simulink model "UDE_quadrotor"  (R2017b)
settings: Solver=ode4  StartTime=0.0  StopTime=40  FixedStep=0.001  RelTol=1e-3
InitFcn:
  | initial_conditions_and_parameters;
values from neighbouring files (symbols this model uses):
  psi_initial = 0.0    (= 0)    [Parameters_and_initial_conditions.m]
  T_passive = 0.5    [Parameters_and_initial_conditions.m]
  theta_initial = 0.0    (= 0)    [Parameters_and_initial_conditions.m]
undefined symbols (not defined in the file or in its folder): a1_x, a1_y, a1_z, a2_x, a2_y, a2_z, CD, Enable_desired_angular_rate_differentiator, ESC_k, ESC_p, f_g, ftau_b, g, hM, hT, Inner_loop_controller_switch, Ir, kd_h, kd_phi, kd_psi, kd_theta, kd_x, kd_y, kd_z, kp_phi, kp_psi, kp_theta, kp_x, kp_y, kp_z, LT, m, p_initial, phi_initial, q_initial, r_initial, T_dif, T_max, T_phi, T_phi1, T_phi2, T_phi3, T_theta, T_theta1, T_theta2, T_theta3, T_x, T_y, T_z, tau_x_max, tau_y_max, tau_z_max, Tf_x, Tf_y, Tf_z, Tn_h, Tn_x, Tn_y, Tn_z, u_initial ... (+5)
libraries: aerolibanim x1, simulink x1, dspsrcs4 x1
(part 1 of 2)
settings Model: Creator=Sky  LastModifiedBy=Sky
settings SolverCC: AlgebraicLoopSolver=LineSearch

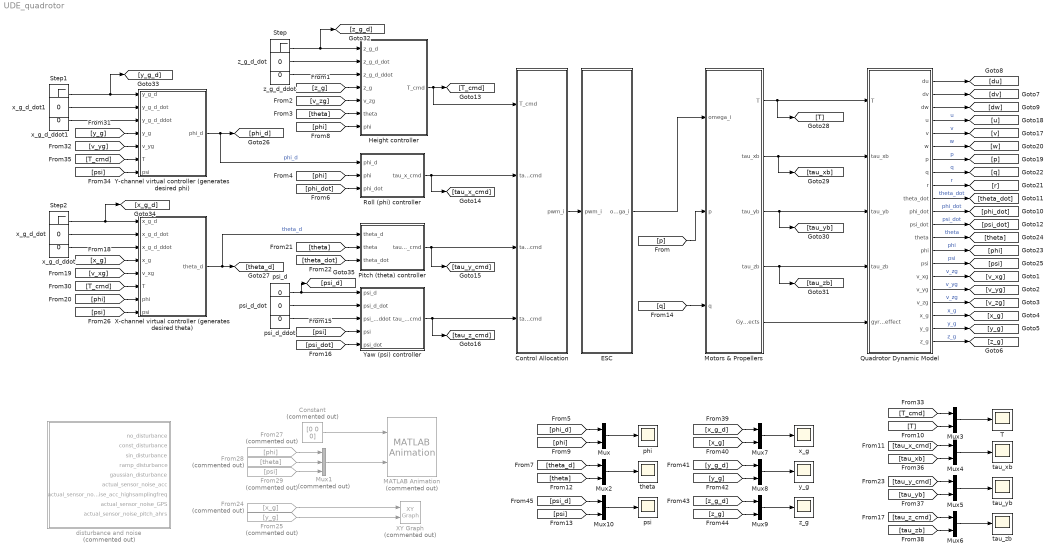
== system UDE_quadrotor ==
  Constant : Constant  Commented=on  Value=[0 0 0]
  Control Allocation : Subsystem
  ESC : Subsystem
  From24 : From  Commented=on  GotoTag=x_g
  From25 : From  Commented=on  GotoTag=y_g
  From27 : From  Commented=on  GotoTag=phi
  From28 : From  Commented=on  GotoTag=theta
  From29 : From  Commented=on  GotoTag=psi
  Height controller : Subsystem
  MATLAB Animation : aerolibanim/MATLAB Animation  Tag=Matlab Animation 6 DOF  Commented=on  Vehicles=1  Geometries='astredwedge.mat'  BoundingBoxCoordinates=[-50,50,-50,50,-50,50]  CameraOffset=[-50,-50,-50]  CameraViewAngle=3  SampleTime=0.2  FigurePosition=[386,218,535,361]
      settings: SourceProductName=Aerospace Blockset  SourceProductBaseCode=AE
  Motors & Propellers : Subsystem
  Mux{,2..10} (10 alike) : Mux  Inputs=2
  Mux1 : Mux  Commented=on  Inputs=3
  Pitch (theta) controller : Subsystem
  Quadrotor Dynamic Model : Subsystem
  Roll (phi) controller : Subsystem
  Step : Step  Time=15  After=-1  SampleTime=0
  Step1 : Step  Time=15  SampleTime=0
  Step2 : Step  Time=15  After=-2  SampleTime=0
  T : Scope
  X-channel virtual controller (generates desired theta) : Subsystem
  XY Graph : simulink/Sinks/XY Graph  Commented=on  xmin=-500  xmax=500  ymin=-500  ymax=500  st=-1
  Y-channel virtual controller (generates desired phi) : Subsystem
  Yaw (psi) controller : Subsystem
  disturbance and noise : Subsystem  Commented=on
  phi : Scope
  psi : Scope
  psi_d : Constant  Value=0
  psi_d_ddot : Constant  Value=0
  psi_d_dot : Constant  Value=0
  tau_xb : Scope
  tau_yb : Scope
  tau_zb : Scope
  theta : Scope
  x_g : Scope
  x_g_d_ddot : Constant  Value=0
  x_g_d_ddot1 : Constant  Value=0
  x_g_d_dot : Constant  Value=0
  x_g_d_dot1 : Constant  Value=0
  y_g : Scope
  z_g : Scope
  z_g_d_ddot : Constant  Value=0
  z_g_d_dot : Constant  Value=0
  wires:
  Height controller/1(T_cmd) -> [T_cmd], Control Allocation/1(T_cmd)
  [v_zg] -> Height controller/5(v_zg)
  [phi] -> Height controller/7(phi)
  [theta] -> Height controller/6(theta)
  [phi] -> Mux/2
  Y-channel virtual controller (generates desired phi)/1(phi_d) -> Roll (phi) controller/1(phi_d), [phi_d]  "phi_d"
  [phi] -> Roll (phi) controller/2(phi)
  [phi_dot] -> Roll (phi) controller/3(phi_dot)
  Step/1 -> [z_g_d], Height controller/1(z_g_d)
  z_g_d_dot/1 -> Height controller/2(z_g_d_dot)
  [T] -> Mux3/2
  [theta] -> Mux2/2
  [theta_dot] -> Pitch (theta) controller/3(theta_dot)
  X-channel virtual controller (generates desired theta)/1(theta_d) -> Pitch (theta) controller/1(theta_d), [theta_d]  "theta_d"
  [theta] -> Pitch (theta) controller/2(theta)
  Constant/1 -> MATLAB Animation/1
  From27/1 -> Mux1/1
  From28/1 -> Mux1/2
  From29/1 -> Mux1/3
  Mux1/1 -> MATLAB Animation/2
  From24/1 -> XY Graph/1
  From25/1 -> XY Graph/2
  [psi] -> Yaw (psi) controller/4(psi)
  psi_d_dot/1 -> Yaw (psi) controller/2(psi_d_dot)
  psi_d/1 -> Yaw (psi) controller/1(psi_d), [psi_d]
  [psi_dot] -> Yaw (psi) controller/5(psi_dot)
  Yaw (psi) controller/1(tau_z_cmd) -> Control Allocation/4(tau_z_cmd), [tau_z_cmd]
  x_g_d_ddot/1 -> X-channel virtual controller (generates desired theta)/3(x_g_d_ddot)
  [z_g] -> Height controller/4(z_g)
  Step2/1 -> [x_g_d], X-channel virtual controller (generates desired theta)/1(x_g_d)
  x_g_d_dot/1 -> X-channel virtual controller (generates desired theta)/2(x_g_d_dot)
  [x_g] -> X-channel virtual controller (generates desired theta)/4(x_g)
  [v_xg] -> X-channel virtual controller (generates desired theta)/5(v_xg)
  [phi] -> X-channel virtual controller (generates desired theta)/7(phi)
  [psi] -> X-channel virtual controller (generates desired theta)/8(psi)
  [T_cmd] -> X-channel virtual controller (generates desired theta)/6(T)
  [T_cmd] -> Y-channel virtual controller (generates desired phi)/6(T)
  [psi] -> Y-channel virtual controller (generates desired phi)/7(psi)
  [v_yg] -> Y-channel virtual controller (generates desired phi)/5(v_yg)
  [y_g] -> Y-channel virtual controller (generates desired phi)/4(y_g)
  x_g_d_dot1/1 -> Y-channel virtual controller (generates desired phi)/2(y_g_d_dot)
  Step1/1 -> [y_g_d], Y-channel virtual controller (generates desired phi)/1(y_g_d)
  x_g_d_ddot1/1 -> Y-channel virtual controller (generates desired phi)/3(y_g_d_ddot)
  [phi_d] -> Mux/1
  Mux/1 -> phi/1
  [theta_d] -> Mux2/1
  Mux2/1 -> theta/1
  z_g_d_ddot/1 -> Height controller/3(z_g_d_ddot)
  psi_d_ddot/1 -> Yaw (psi) controller/3(psi_d_ddot)
  Roll (phi) controller/1(tau_x_cmd) -> Control Allocation/2(tau_x_cmd), [tau_x_cmd]
  ESC/1(omega_i) -> Motors & Propellers/1(omega_i)
  Control Allocation/1(pwm_i) -> ESC/1(pwm_i)
  [q] -> Motors & Propellers/3(q)
  [p] -> Motors & Propellers/2(p)
  Motors & Propellers/1(T) -> Quadrotor Dynamic Model/1(T), [T]
  Motors & Propellers/2(tau_xb) -> Quadrotor Dynamic Model/2(tau_xb), [tau_xb]
  Motors & Propellers/3(tau_yb) -> Quadrotor Dynamic Model/3(tau_yb), [tau_yb]
  [T_cmd] -> Mux3/1
  Mux3/1 -> T/1
  Pitch (theta) controller/1(tau_y_cmd) -> Control Allocation/3(tau_y_cmd), [tau_y_cmd]
  Motors & Propellers/4(tau_zb) -> Quadrotor Dynamic Model/4(tau_zb), [tau_zb]
  Mux4/1 -> tau_xb/1
  [tau_x_cmd] -> Mux4/1
  [tau_xb] -> Mux4/2
  [tau_yb] -> Mux5/2
  [tau_y_cmd] -> Mux5/1
  Mux5/1 -> tau_yb/1
  [tau_zb] -> Mux6/2
  [tau_z_cmd] -> Mux6/1
  Mux6/1 -> tau_zb/1
  Mux7/1 -> x_g/1
  [x_g_d] -> Mux7/1
  [x_g] -> Mux7/2
  [y_g] -> Mux8/2
  [y_g_d] -> Mux8/1
  Mux8/1 -> y_g/1
  Mux9/1 -> z_g/1
  [z_g_d] -> Mux9/1
  [z_g] -> Mux9/2
  Mux10/1 -> psi/1
  [psi] -> Mux10/2
  [psi_d] -> Mux10/1
  Quadrotor Dynamic Model/3(dw) -> [dw]
  Quadrotor Dynamic Model/8(q) -> [q]  "q"
  Quadrotor Dynamic Model/12(psi_dot) -> [psi_dot]  "psi_dot"
  Quadrotor Dynamic Model/18(v_zg) -> [v_zg]  "v_zg"
  Quadrotor Dynamic Model/5(v) -> [v]  "v"
  Quadrotor Dynamic Model/9(r) -> [r]  "r"
  Quadrotor Dynamic Model/11(phi_dot) -> [phi_dot]  "phi_dot"
  Quadrotor Dynamic Model/1(du) -> [du]
  Quadrotor Dynamic Model/19(x_g) -> [x_g]  "x_g"
  Quadrotor Dynamic Model/20(y_g) -> [y_g]  "y_g"
  Quadrotor Dynamic Model/16(v_xg) -> [v_xg]  "v_zg"
  Quadrotor Dynamic Model/15(psi) -> [psi]  "psi"
  Quadrotor Dynamic Model/4(u) -> [u]  "u"
  Quadrotor Dynamic Model/13(theta) -> [theta]  "theta"
  Quadrotor Dynamic Model/17(v_yg) -> [v_yg]  "v_yg"
  Quadrotor Dynamic Model/14(phi) -> [phi]  "phi"
  Quadrotor Dynamic Model/21(z_g) -> [z_g]  "z_g"
  Quadrotor Dynamic Model/6(w) -> [w]  "w"
  Quadrotor Dynamic Model/7(p) -> [p]  "p"
  Quadrotor Dynamic Model/2(dv) -> [dv]
  Quadrotor Dynamic Model/10(theta_dot) -> [theta_dot]  "theta_dot"
  Motors & Propellers/5(Gyroscopic effects) -> Quadrotor Dynamic Model/5(gyroeffect)

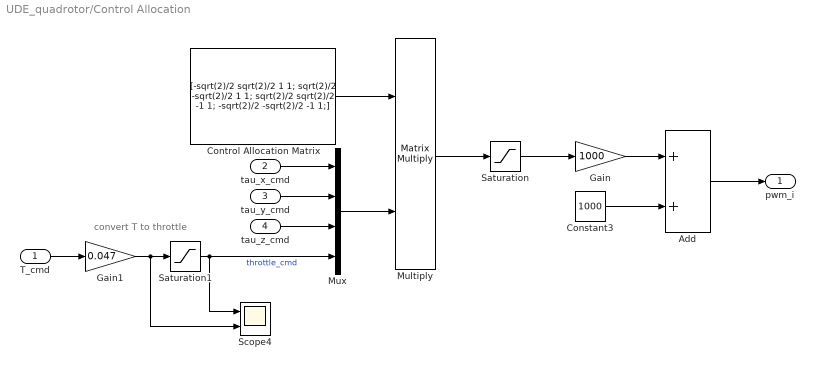
== system UDE_quadrotor/Control Allocation ==
  note: convert T to throttle
  T_cmd : Inport
  tau_x_cmd : Inport  Port=2
  tau_y_cmd : Inport  Port=3
  tau_z_cmd : Inport  Port=4
  Add : Sum
  Constant3 : Constant  Value=1000
  Control Allocation Matrix : Constant  Value="[-sqrt(2)/2  sqrt(2)/2  1 1; sqrt(2)/2 -sqrt(2)/2  1 1; sqrt(2)/2  sqrt(2)/2 -1 1; -sqrt(2)/2 -sqrt(2)/2 -1 1;]"
  Gain : Gain  Gain=1000  OutDataTypeStr=Inherit: Same as input
  Gain1 : Gain  Gain=0.047
  Multiply : Product  Multiplication=Matrix(*)  OutDataTypeStr=Inherit: Same as first input
  Mux : Mux
  Saturation : Saturate  UpperLimit=1  LowerLimit=0
  Saturation1 : Saturate  UpperLimit=1  LowerLimit=0
  Scope4 : Scope  NumInputPorts=2
  pwm_i : Outport
  wires:
  Constant3/1 -> Add/2
  Saturation/1 -> Gain/1
  Saturation1/1 -> Scope4/1, Mux/4  "throttle_cmd"
  tau_y_cmd/1 -> Mux/2
  Add/1 -> pwm_i/1
  Multiply/1 -> Saturation/1
  Gain/1 -> Add/1
  tau_x_cmd/1 -> Mux/1
  tau_z_cmd/1 -> Mux/3
  Mux/1 -> Multiply/2
  Control Allocation Matrix/1 -> Multiply/1
  Gain1/1 -> Scope4/2, Saturation1/1
  T_cmd/1 -> Gain1/1

== system UDE_quadrotor/ESC ==
  pwm_i : Inport
  Add : Sum  AccumDataTypeStr=double
  Constant : Constant  Value=ESC_p
  Constant3 : Constant  Value=1000  OutDataTypeStr=double
  Gain : Gain  Gain=0.001  OutDataTypeStr=Inherit: Same as input
  Gain1 : Gain  Gain=ESC_k  OutDataTypeStr=Inherit: Same as input
  Saturation : Saturate  UpperLimit=2000  LowerLimit=1000
  Sum : Sum  Inputs=|+-
  omega_i : Outport
  wires:
  Constant3/1 -> Sum/2
  pwm_i/1 -> Saturation/1
  Saturation/1 -> Sum/1
  Sum/1 -> Gain/1
  Constant/1 -> Add/2
  Gain/1 -> Gain1/1
  Gain1/1 -> Add/1
  Add/1 -> omega_i/1

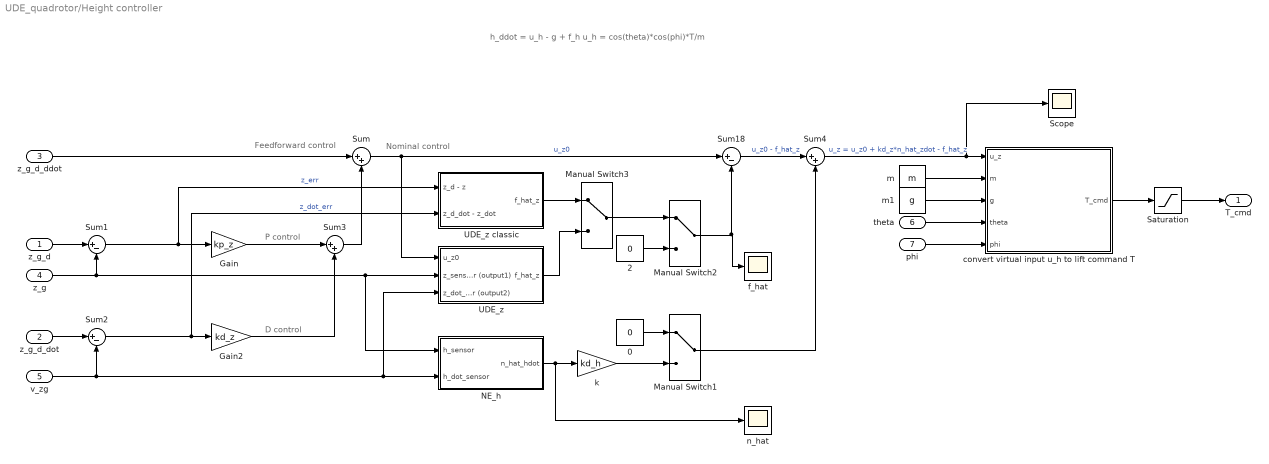
== system UDE_quadrotor/Height controller ==
  note: P control
  note: h_ddot = u_h - g + f_h
      | u_h = cos(theta)*cos(phi)*T/m
  note: D control
  note: Feedforward control
  note: Nominal control
  z_g_d : Inport
  z_g_d_dot : Inport  Port=2
  z_g_d_ddot : Inport  Port=3
  z_g : Inport  Port=4
  v_zg : Inport  Port=5
  theta : Inport  Port=6
  phi : Inport  Port=7
  0 : Constant  Value=0
  2 : Constant  Value=0
  Gain : Gain  Gain=kp_z
  Gain2 : Gain  Gain=kd_z
  Manual Switch1 : ManualSwitch
  Manual Switch2 : ManualSwitch
  Manual Switch3 : ManualSwitch
  NE_h : Subsystem
  Saturation : Saturate  UpperLimit=T_max  LowerLimit=0
  Scope : Scope
  Sum : Sum  Inputs=|++
  Sum1 : Sum  Inputs=|+-
  Sum18 : Sum  Inputs=|+-
  Sum2 : Sum  Inputs=|+-
  Sum3 : Sum  Inputs=|++
  Sum4 : Sum  Inputs=|++
  UDE_z : Subsystem
  UDE_z classic : Subsystem
  convert virtual input u_h to lift command T : MATLAB Function  TreatAsAtomicUnit=on
  f_hat : Scope
  k : Gain  Gain=kd_h
  m : Constant  Value=m
  m1 : Constant  Value=g
  n_hat : Scope
  T_cmd : Outport
  wires:
  z_g_d_dot/1 -> Sum2/1
  Sum3/1 -> Sum/2
  Sum/1 -> Sum18/1, UDE_z/1(u_z0)  "u_z0"
  Gain/1 -> Sum3/1
  z_g_d/1 -> Sum1/1
  Sum1/1 -> UDE_z classic/1(z_d - z), Gain/1  "z_err"
  Sum2/1 -> UDE_z classic/2(z_d_dot - z_dot), Gain2/1  "z_dot_err"
  Gain2/1 -> Sum3/2
  Manual Switch3/1 -> Manual Switch2/1
  Sum18/1 -> Sum4/1  "u_z0 - f_hat_z"
  k/1 -> Manual Switch1/2
  NE_h/1(n_hat_hdot) -> n_hat/1, k/1
  0/1 -> Manual Switch1/1
  Manual Switch1/1 -> Sum4/2
  Manual Switch2/1 -> f_hat/1, Sum18/2
  Sum4/1 -> Scope/1, convert virtual input u_h to lift command T/1(u_z)  "u_z = u_z0 + kd_z*n_hat_zdot - f_hat_z"
  phi/1 -> convert virtual input u_h to lift command T/5(phi)
  m/1 -> convert virtual input u_h to lift command T/2(m)
  theta/1 -> convert virtual input u_h to lift command T/4(theta)
  z_g/1 -> NE_h/1(h_sensor), UDE_z/2(z_sensor (output1)), Sum1/2
  v_zg/1 -> NE_h/2(h_dot_sensor), UDE_z/3(z_dot_sensor (output2)), Sum2/2
  convert virtual input u_h to lift command T/1(T_cmd) -> Saturation/1
  UDE_z/1(f_hat_z) -> Manual Switch3/2
  z_g_d_ddot/1 -> Sum/1
  Saturation/1 -> T_cmd/1
  m1/1 -> convert virtual input u_h to lift command T/3(g)
  UDE_z classic/1(f_hat_z) -> Manual Switch3/1
  2/1 -> Manual Switch2/2

== system UDE_quadrotor/Motors & Propellers ==
  omega_i : Inport
  p : Inport  Port=2
  q : Inport  Port=3
  Demux : Demux  Outputs=3
  Force : Subsystem
  Gyroscopic_Torque : Subsystem
  Rotor_Generated_Torque : Subsystem
  T : Outport
  tau_xb : Outport  Port=2
  tau_yb : Outport  Port=3
  tau_zb : Outport  Port=4
  Gyroscopic effects : Outport  Port=5
  wires:
  Rotor_Generated_Torque/1(Torque) -> Demux/1
  p/1 -> Gyroscopic_Torque/2(p)
  omega_i/1 -> Force/1(Rotor_speed), Gyroscopic_Torque/1(Rotor_speed), Rotor_Generated_Torque/1(Rotor_speed)
  Force/1(force_B_N) -> T/1
  Gyroscopic_Torque/1(gyroscopic_torque) -> Gyroscopic effects/1
  Demux/1 -> tau_xb/1
  Demux/2 -> tau_yb/1
  Demux/3 -> tau_zb/1
  q/1 -> Gyroscopic_Torque/3(q)

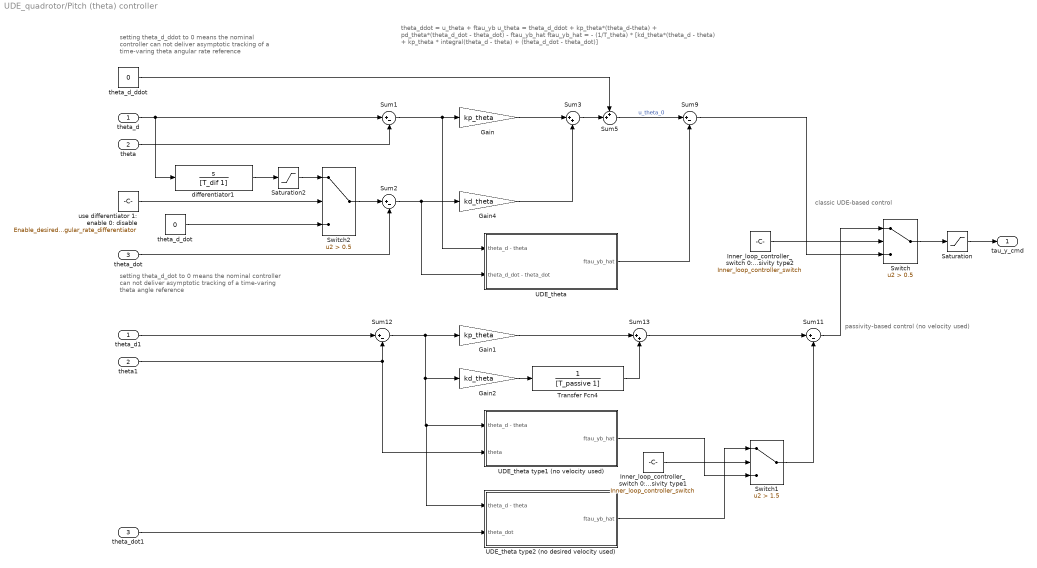
== system UDE_quadrotor/Pitch (theta) controller ==
  note: setting theta_d_ddot to 0 means the nominal controller can not deliver asymptotic tracking of a time-varing theta angular rate reference
  note: setting theta_d_dot to 0 means the nominal controller can not deliver asymptotic tracking of a time-varing theta angle reference
  note: theta_ddot = u_theta + ftau_yb
      | u_theta = theta_d_ddot + kp_theta*(theta_d-theta) + pd_theta*(theta_d_dot - theta_dot) - ftau_yb_hat
      | ftau_yb_hat = - (1/T_theta) * [kd_theta*(theta_d - theta) + kp_theta * integral(theta_d - theta) + (theta_d_dot - theta_dot)]
  note: classic UDE-based control
  note: passivity-based control (no velocity used)
  theta_d : Inport
  theta : Inport  Port=2
  theta_dot : Inport  Port=3
  Gain : Gain  Gain=kp_theta
  Gain1 : Gain  Gain=kp_theta
  Gain2 : Gain  Gain=kd_theta
  Gain4 : Gain  Gain=kd_theta
  Inner_loop_controller_switch 0: classic UDE 1: passivity type1 2: passivity type1 : Constant  Value=Inner_loop_controller_switch
  Inner_loop_controller_switch 0: classic UDE 1: passivity type1 2: passivity type2 : Constant  Value=Inner_loop_controller_switch
  Saturation : Saturate  UpperLimit=tau_y_max  LowerLimit=-tau_y_max
  Saturation2 : Saturate  UpperLimit=0.05  LowerLimit=-0.05
  Sum{1..2,9,11..12} (5 alike) : Sum  Inputs=|+-
  Sum13 : Sum  Inputs=|++
  Sum3 : Sum  Inputs=|++
  Sum5 : Sum  Inputs=++|
  Switch : Switch  Criteria=u2 > Threshold  Threshold=0.5
  Switch1 : Switch  Criteria=u2 > Threshold  Threshold=1.5
  Switch2 : Switch  Criteria=u2 > Threshold  Threshold=0.5
  Transfer Fcn4 : TransferFcn  Denominator=[T_passive 1]
  UDE_theta : Subsystem
  UDE_theta type1 (no velocity used) : Subsystem
  UDE_theta type2 (no desired velocity used) : Subsystem
  differentiator1 : TransferFcn  Numerator=[1 0]  Denominator=[T_dif 1]
  theta1 : InportShadow  Port=2
  theta_d1 : InportShadow
  theta_d_ddot : Constant  Value=0
  theta_d_dot : Constant  Value=0
  theta_dot1 : InportShadow  Port=3
  "use differentiator 1: enable 0: disable " : Constant  Value=Enable_desired_angular_rate_differentiator
  tau_y_cmd : Outport
  wires:
  theta_d/1 -> differentiator1/1, Sum1/1
  theta_dot/1 -> Sum2/2
  Gain/1 -> Sum3/1
  theta/1 -> Sum1/2
  Gain4/1 -> Sum3/2
  Switch2/1 -> Sum2/1
  theta_d_ddot/1 -> Sum5/1
  Sum3/1 -> Sum5/2
  Sum2/1 -> UDE_theta/2(theta_d_dot - theta_dot), Gain4/1
  Sum1/1 -> UDE_theta/1(theta_d - theta), Gain/1
  Inner_loop_controller_switch 0: classic UDE 1: passivity type1 2: passivity type2/1 -> Switch/2
  Switch/1 -> Saturation/1
  Gain2/1 -> Transfer Fcn4/1
  Transfer Fcn4/1 -> Sum13/2
  Gain1/1 -> Sum13/1
  Sum11/1 -> Switch/1
  Sum9/1 -> Switch/3
  UDE_theta type1 (no velocity used)/1(ftau_yb_hat) -> Switch1/3
  theta1/1 -> UDE_theta type1 (no velocity used)/2(theta), Sum12/2
  Sum12/1 -> Gain1/1, UDE_theta type2 (no desired velocity used)/1(theta_d - theta), UDE_theta type1 (no velocity used)/1(theta_d - theta), Gain2/1
  Sum13/1 -> Sum11/1
  Sum5/1 -> Sum9/1  "u_theta_0"
  UDE_theta/1(ftau_yb_hat) -> Sum9/2
  theta_d1/1 -> Sum12/1
  theta_d_dot/1 -> Switch2/3
  Saturation/1 -> tau_y_cmd/1
  differentiator1/1 -> Saturation2/1
  "use differentiator 1: enable 0: disable "/1 -> Switch2/2
  UDE_theta type2 (no desired velocity used)/1(ftau_yb_hat) -> Switch1/1
  Switch1/1 -> Sum11/2
  theta_dot1/1 -> UDE_theta type2 (no desired velocity used)/2(theta_dot)
  Saturation2/1 -> Switch2/1
  Inner_loop_controller_switch 0: classic UDE 1: passivity type1 2: passivity type1/1 -> Switch1/2

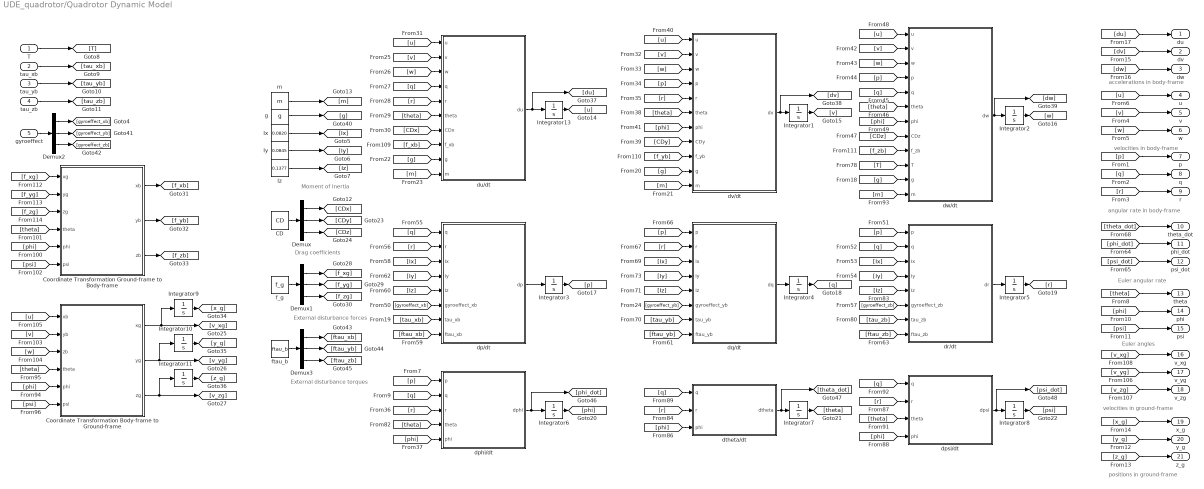
== system UDE_quadrotor/Quadrotor Dynamic Model ==
  note: velocities in body-frame
  note: accelerations in body-frame
  note: Moment of Inertia
  note: Drag coefficients
  note: External disturbance forces
  note: External disturbance torques
  note: angular rate in body-frame
  note: Euler angular rate
  note: Euler angles
  note: velocities in ground-frame
  note: positions in ground-frame
  T : Inport
  tau_xb : Inport  Port=2
  tau_yb : Inport  Port=3
  tau_zb : Inport  Port=4
  gyroeffect : Inport  Port=5
  CD : Constant  Value=CD
  Coordinate Transformation Body-frame to Ground-frame : MATLAB Function  TreatAsAtomicUnit=on
  Coordinate Transformation Ground-frame to Body-frame : MATLAB Function  TreatAsAtomicUnit=on
  Demux{,1..3} (4 alike) : Demux  Outputs=3
  Integrator1 : Integrator  InitialCondition=v_initial
  Integrator10 : Integrator  InitialCondition=y_g_initial
  Integrator11 : Integrator  InitialCondition=z_g_initial
  Integrator13 : Integrator  InitialCondition=u_initial
  Integrator2 : Integrator  InitialCondition=w_initial
  Integrator3 : Integrator  InitialCondition=p_initial
  Integrator4 : Integrator  InitialCondition=q_initial
  Integrator5 : Integrator  InitialCondition=r_initial
  Integrator6 : Integrator  InitialCondition=phi_initial
  Integrator7 : Integrator  InitialCondition=theta_initial
  Integrator8 : Integrator  InitialCondition=psi_initial
  Integrator9 : Integrator  InitialCondition=x_g_initial
  Ix : Constant  Value=0.0820
  Iy : Constant  Value=0.0845
  Iz : Constant  Value=0.1377
  dp/dt : MATLAB Function  TreatAsAtomicUnit=on
  dphi/dt : MATLAB Function  TreatAsAtomicUnit=on
  dpsi/dt : MATLAB Function  TreatAsAtomicUnit=on
  dq/dt : MATLAB Function  TreatAsAtomicUnit=on
  dr/dt : MATLAB Function  TreatAsAtomicUnit=on
  dtheta/dt : MATLAB Function  TreatAsAtomicUnit=on
  du/dt : MATLAB Function  TreatAsAtomicUnit=on
  dv/dt : MATLAB Function  TreatAsAtomicUnit=on
  dw/dt : MATLAB Function  TreatAsAtomicUnit=on
  f_g : Constant  Value=f_g
  ftau_b : Constant  Value=ftau_b
  g : Constant  Value=g
  m : Constant  Value=m
  du : Outport
  dv : Outport  Port=2
  dw : Outport  Port=3
  u : Outport  Port=4
  v : Outport  Port=5
  w : Outport  Port=6
  p : Outport  Port=7
  q : Outport  Port=8
  r : Outport  Port=9
  theta_dot : Outport  Port=10
  phi_dot : Outport  Port=11
  psi_dot : Outport  Port=12
  theta : Outport  Port=13
  phi : Outport  Port=14
  psi : Outport  Port=15
  v_xg : Outport  Port=16
  v_yg : Outport  Port=17
  v_zg : Outport  Port=18
  x_g : Outport  Port=19
  y_g : Outport  Port=20
  z_g : Outport  Port=21
  wires:
  Ix/1 -> [Ix]
  Iy/1 -> [Iy]
  Iz/1 -> [Iz]
  T/1 -> [T]
  tau_xb/1 -> [tau_xb]
  tau_yb/1 -> [tau_yb]
  tau_zb/1 -> [tau_zb]
  CD/1 -> Demux/1
  m/1 -> [m]
  [v] -> du/dt/2(v)
  [w] -> du/dt/3(w)
  [q] -> du/dt/4(q)
  [r] -> du/dt/5(r)
  [theta] -> du/dt/6(theta)
  [CDx] -> du/dt/7(CDx)
  [u] -> du/dt/1(u)
  du/dt/1(du) -> [du], Integrator13/1
  Integrator13/1 -> [u]
  [v] -> dv/dt/2(v)
  [w] -> dv/dt/3(w)
  [p] -> dv/dt/4(p)
  [r] -> dv/dt/5(r)
  [theta] -> dv/dt/6(theta)
  [CDy] -> dv/dt/8(CDy)
  [u] -> dv/dt/1(u)
  dv/dt/1(dv) -> [dv], Integrator1/1
  Integrator1/1 -> [v]
  [phi] -> dv/dt/7(phi)
  [v] -> dw/dt/2(v)
  [w] -> dw/dt/3(w)
  [p] -> dw/dt/4(p)
  [q] -> dw/dt/5(q)
  [theta] -> dw/dt/6(theta)
  [CDz] -> dw/dt/8(CDz)
  [u] -> dw/dt/1(u)
  dw/dt/1(dw) -> [dw], Integrator2/1
  Integrator2/1 -> [w]
  [phi] -> dw/dt/7(phi)
  dp/dt/1(dp) -> Integrator3/1
  Integrator3/1 -> [p]
  [gyroeffect_xb] -> dp/dt/6(gyroeffect_xb)
  [q] -> dp/dt/1(q)
  [r] -> dp/dt/2(r)
  [Iz] -> dp/dt/5(Iz)
  [Ix] -> dp/dt/3(Ix)
  [Iy] -> dp/dt/4(Iy)
  dq/dt/1(dq) -> Integrator4/1
  Integrator4/1 -> [q]
  [p] -> dq/dt/1(p)
  [r] -> dq/dt/2(r)
  [Iz] -> dq/dt/5(Iz)
  [Ix] -> dq/dt/3(Ix)
  [tau_yb] -> dq/dt/7(tau_yb)
  [Iy] -> dq/dt/4(Iy)
  dr/dt/1(dr) -> Integrator5/1
  Integrator5/1 -> [r]
  [tau_zb] -> dr/dt/7(tau_zb)
  [Iz] -> dr/dt/5(Iz)
  dphi/dt/1(dphi) -> [phi_dot], Integrator6/1
  Integrator6/1 -> [phi]
  [p] -> dphi/dt/1(p)
  [q] -> dphi/dt/2(q)
  [r] -> dphi/dt/3(r)
  [theta] -> dphi/dt/4(theta)
  [phi] -> dphi/dt/5(phi)
  dtheta/dt/1(dtheta) -> [theta_dot], Integrator7/1
  Integrator7/1 -> [theta]
  [q] -> dtheta/dt/1(q)
  [r] -> dtheta/dt/2(r)
  [phi] -> dtheta/dt/3(phi)
  dpsi/dt/1(dpsi) -> [psi_dot], Integrator8/1
  Integrator8/1 -> [psi]
  [q] -> dpsi/dt/1(q)
  [r] -> dpsi/dt/2(r)
  [theta] -> dpsi/dt/3(theta)
  [phi] -> dpsi/dt/4(phi)
  Demux/1 -> [CDx]
  Demux/2 -> [CDy]
  Demux/3 -> [CDz]
  [u] -> u/1
  [v] -> v/1
  [w] -> w/1
  [p] -> p/1
  [q] -> q/1
  [r] -> r/1
  [theta] -> theta/1
  [phi] -> phi/1
  [psi] -> psi/1
  [T] -> dw/dt/10(T)
  [m] -> dw/dt/12(m)
  [theta] -> Coordinate Transformation Body-frame to Ground-frame/4(theta)
  [phi] -> Coordinate Transformation Body-frame to Ground-frame/5(phi)
  [psi] -> Coordinate Transformation Body-frame to Ground-frame/6(psi)
  [theta] -> Coordinate Transformation Ground-frame to Body-frame/4(theta)
  [phi] -> Coordinate Transformation Ground-frame to Body-frame/5(phi)
  [psi] -> Coordinate Transformation Ground-frame to Body-frame/6(psi)
  [u] -> Coordinate Transformation Body-frame to Ground-frame/1(xb)
  [v] -> Coordinate Transformation Body-frame to Ground-frame/2(yb)
  [w] -> Coordinate Transformation Body-frame to Ground-frame/3(zb)
  Coordinate Transformation Body-frame to Ground-frame/1(xg) -> Integrator9/1, [v_xg]
  Coordinate Transformation Body-frame to Ground-frame/2(yg) -> Integrator10/1, [v_yg]
  Coordinate Transformation Body-frame to Ground-frame/3(zg) -> Integrator11/1, [v_zg]
  [v_xg] -> v_xg/1
  [v_yg] -> v_yg/1
  [v_zg] -> v_zg/1
  f_g/1 -> Demux1/1
  Demux1/1 -> [f_xg]
  Demux1/2 -> [f_yg]
  Demux1/3 -> [f_zg]
  Coordinate Transformation Ground-frame to Body-frame/1(xb) -> [f_xb]
  Coordinate Transformation Ground-frame to Body-frame/2(yb) -> [f_yb]
  Coordinate Transformation Ground-frame to Body-frame/3(zb) -> [f_zb]
  [f_xb] -> du/dt/8(f_xb)
  [f_yb] -> dv/dt/9(f_yb)
  [f_zb] -> dw/dt/9(f_zb)
  [f_xg] -> Coordinate Transformation Ground-frame to Body-frame/1(xg)
  [f_yg] -> Coordinate Transformation Ground-frame to Body-frame/2(yg)
  [f_zg] -> Coordinate Transformation Ground-frame to Body-frame/3(zg)
  Integrator9/1 -> [x_g]
  Integrator10/1 -> [y_g]
  Integrator11/1 -> [z_g]
  [x_g] -> x_g/1
  [y_g] -> y_g/1
  [z_g] -> z_g/1
  [du] -> du/1
  [dv] -> dv/1
  [dw] -> dw/1
  g/1 -> [g]
  [g] -> dw/dt/11(g)
  [g] -> dv/dt/10(g)
  [m] -> dv/dt/11(m)
  [m] -> du/dt/10(m)
  [g] -> du/dt/9(g)
  Demux2/3 -> [gyroeffect_zb]
  Demux2/2 -> [gyroeffect_yb]
  Demux2/1 -> [gyroeffect_xb]
  gyroeffect/1 -> Demux2/1
  [tau_xb] -> dp/dt/7(tau_xb)
  [gyroeffect_yb] -> dq/dt/6(gyroeffect_yb)
  [Iy] -> dr/dt/4(Iy)
  [p] -> dr/dt/1(p)
  [q] -> dr/dt/2(q)
  [Ix] -> dr/dt/3(Ix)
  [gyroeffect_zb] -> dr/dt/6(gyroeffect_zb)
  Demux3/3 -> [ftau_zb]
  Demux3/1 -> [ftau_xb]
  Demux3/2 -> [ftau_yb]
  ftau_b/1 -> Demux3/1
  [ftau_xb] -> dp/dt/8(ftau_xb)
  [ftau_yb] -> dq/dt/8(ftau_yb)
  [ftau_zb] -> dr/dt/8(ftau_zb)
  [theta_dot] -> theta_dot/1
  [phi_dot] -> phi_dot/1
  [psi_dot] -> psi_dot/1

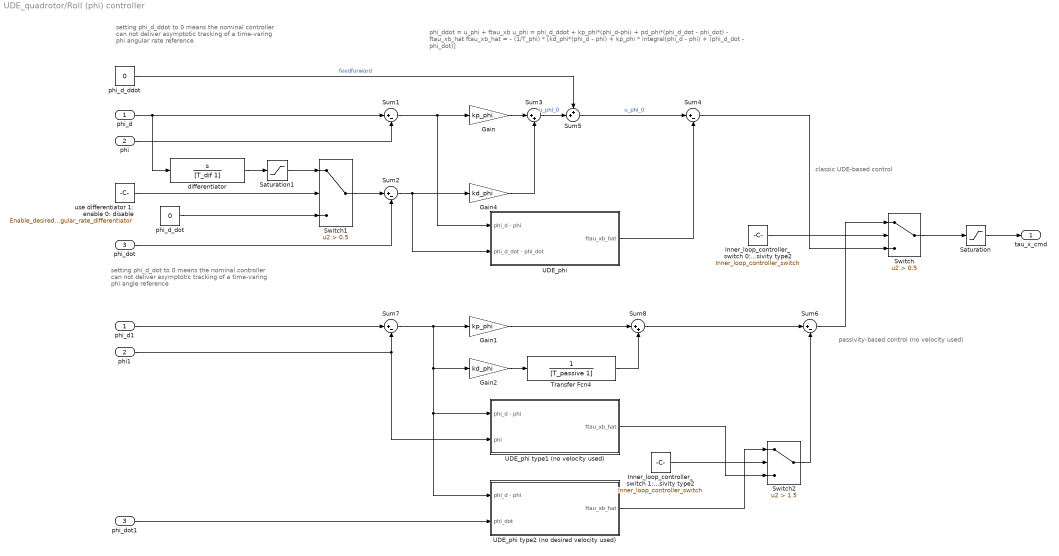
== system UDE_quadrotor/Roll (phi) controller ==
  note: passivity-based control (no velocity used)
  note: phi_ddot = u_phi + ftau_xb
      | u_phi = phi_d_ddot + kp_phi*(phi_d-phi) + pd_phi*(phi_d_dot - phi_dot) - ftau_xb_hat
      | ftau_xb_hat = - (1/T_phi) * [kd_phi*(phi_d - phi) + kp_phi * integral(phi_d - phi) + (phi_d_dot - phi_dot)]
  note: setting phi_d_ddot to 0 means the nominal controller can not deliver asymptotic tracking of a time-varing phi angular rate reference
  note: setting phi_d_dot to 0 means the nominal controller can not deliver asymptotic tracking of a time-varing phi angle reference
  note: classic UDE-based control
  phi_d : Inport
  phi : Inport  Port=2
  phi_dot : Inport  Port=3
  Gain : Gain  Gain=kp_phi
  Gain1 : Gain  Gain=kp_phi
  Gain2 : Gain  Gain=kd_phi
  Gain4 : Gain  Gain=kd_phi
  Inner_loop_controller_switch 0: classic UDE 1: passivity type1 2: passivity type2 : Constant  Value=Inner_loop_controller_switch
  Inner_loop_controller_switch 1: passivity type1 2: passivity type2 : Constant  Value=Inner_loop_controller_switch
  Saturation : Saturate  UpperLimit=tau_x_max  LowerLimit=-tau_x_max
  Saturation1 : Saturate  UpperLimit=0.05  LowerLimit=-0.05
  Sum{1..2,4,6..7} (5 alike) : Sum  Inputs=|+-
  Sum3 : Sum  Inputs=|++
  Sum5 : Sum  Inputs=++|
  Sum8 : Sum  Inputs=|++
  Switch : Switch  Criteria=u2 > Threshold  Threshold=0.5
  Switch1 : Switch  Criteria=u2 > Threshold  Threshold=0.5
  Switch2 : Switch  Criteria=u2 > Threshold  Threshold=1.5
  Transfer Fcn4 : TransferFcn  Denominator=[T_passive 1]
  UDE_phi : Subsystem
  UDE_phi type1 (no velocity used) : Subsystem
  UDE_phi type2 (no desired velocity used) : Subsystem
  differentiator : TransferFcn  Numerator=[1 0]  Denominator=[T_dif 1]
  phi1 : InportShadow  Port=2
  phi_d1 : InportShadow
  phi_d_ddot : Constant  Value=0
  phi_d_dot : Constant  Value=0
  phi_dot1 : InportShadow  Port=3
  "use differentiator 1: enable 0: disable " : Constant  Value=Enable_desired_angular_rate_differentiator
  tau_x_cmd : Outport
  wires:
  Sum2/1 -> Gain4/1, UDE_phi/2(phi_d_dot - phi_dot)
  phi_dot/1 -> Sum2/2
  Sum1/1 -> Gain/1, UDE_phi/1(phi_d - phi)
  Gain/1 -> Sum3/1
  Sum5/1 -> Sum4/1  "u_phi_0"
  phi/1 -> Sum1/2
  UDE_phi/1(ftau_xb_hat) -> Sum4/2
  Sum4/1 -> Switch/3
  Gain4/1 -> Sum3/2
  UDE_phi type1 (no velocity used)/1(ftau_xb_hat) -> Switch2/3
  phi_d_ddot/1 -> Sum5/1  "feedforward"
  Sum3/1 -> Sum5/2  "u_phi_0"
  phi1/1 -> UDE_phi type1 (no velocity used)/2(phi), Sum7/2
  phi_d1/1 -> Sum7/1
  Gain1/1 -> Sum8/1
  Gain2/1 -> Transfer Fcn4/1
  Sum8/1 -> Sum6/1
  Sum6/1 -> Switch/1
  Switch/1 -> Saturation/1
  Transfer Fcn4/1 -> Sum8/2
  Inner_loop_controller_switch 0: classic UDE 1: passivity type1 2: passivity type2/1 -> Switch/2
  phi_d_dot/1 -> Switch1/3
  differentiator/1 -> Saturation1/1
  Switch1/1 -> Sum2/1
  phi_d/1 -> Sum1/1, differentiator/1
  "use differentiator 1: enable 0: disable "/1 -> Switch1/2
  Saturation/1 -> tau_x_cmd/1
  phi_dot1/1 -> UDE_phi type2 (no desired velocity used)/2(phi_dot)
  Sum7/1 -> UDE_phi type2 (no desired velocity used)/1(phi_d - phi), UDE_phi type1 (no velocity used)/1(phi_d - phi), Gain2/1, Gain1/1
  Switch2/1 -> Sum6/2
  Saturation1/1 -> Switch1/1
  Inner_loop_controller_switch 1: passivity type1 2: passivity type2/1 -> Switch2/2
  UDE_phi type2 (no desired velocity used)/1(ftau_xb_hat) -> Switch2/1

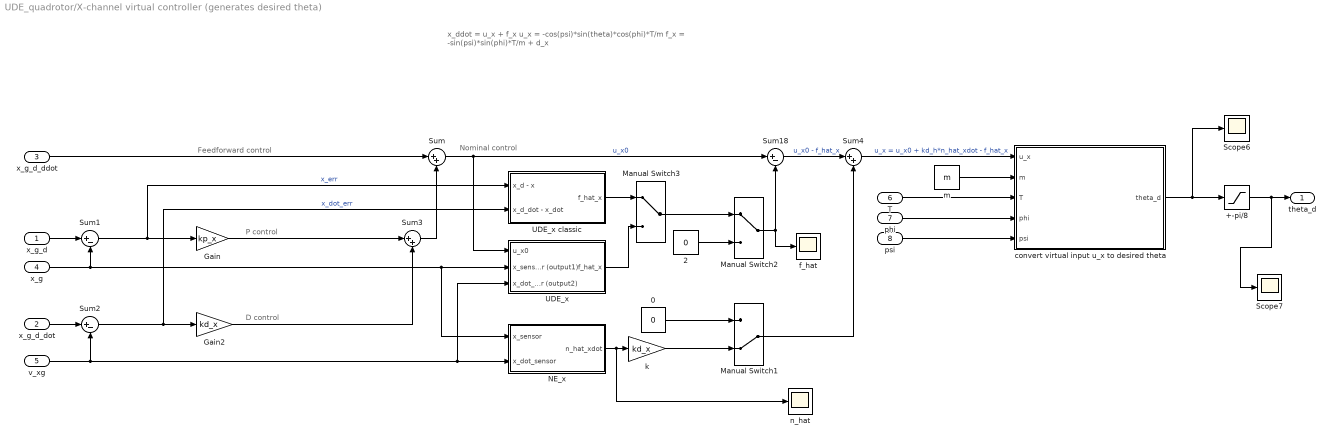
== system UDE_quadrotor/X-channel virtual controller (generates desired theta) ==
  note: P control
  note: x_ddot = u_x + f_x
      | u_x = -cos(psi)*sin(theta)*cos(phi)*T/m
      | f_x = -sin(psi)*sin(phi)*T/m + d_x
  note: D control
  note: Feedforward control
  note: Nominal control
  x_g_d : Inport
  x_g_d_dot : Inport  Port=2
  x_g_d_ddot : Inport  Port=3
  x_g : Inport  Port=4
  v_xg : Inport  Port=5
  T : Inport  Port=6
  phi : Inport  Port=7
  psi : Inport  Port=8
  +-pi/8 : Saturate  UpperLimit=pi/8  LowerLimit=-pi/8
  0 : Constant  Value=0
  2 : Constant  Value=0
  Gain : Gain  Gain=kp_x
  Gain2 : Gain  Gain=kd_x
  Manual Switch1 : ManualSwitch  CurrentSetting=0
  Manual Switch2 : ManualSwitch
  Manual Switch3 : ManualSwitch
  NE_x : Subsystem
  Scope6 : Scope
  Scope7 : Scope
  Sum : Sum  Inputs=|++
  Sum1 : Sum  Inputs=|+-
  Sum18 : Sum  Inputs=|+-
  Sum2 : Sum  Inputs=|+-
  Sum3 : Sum  Inputs=|++
  Sum4 : Sum  Inputs=|++
  UDE_x : Subsystem
  UDE_x classic : Subsystem
  convert virtual input u_x to desired theta : MATLAB Function  TreatAsAtomicUnit=on
  f_hat : Scope
  k : Gain  Gain=kd_x
  m : Constant  Value=m
  n_hat : Scope
  theta_d : Outport
  wires:
  x_g_d_dot/1 -> Sum2/1
  Sum3/1 -> Sum/2
  Sum/1 -> Sum18/1, UDE_x/1(u_x0)  "u_x0"
  Gain/1 -> Sum3/1
  x_g_d/1 -> Sum1/1
  Sum1/1 -> UDE_x classic/1(x_d - x), Gain/1  "x_err"
  Sum2/1 -> UDE_x classic/2(x_d_dot - x_dot), Gain2/1  "x_dot_err"
  Sum18/1 -> Sum4/1  "u_x0 - f_hat_x"
  k/1 -> Manual Switch1/2
  NE_x/1(n_hat_xdot) -> n_hat/1, k/1
  0/1 -> Manual Switch1/1
  Manual Switch1/1 -> Sum4/2
  Manual Switch2/1 -> Sum18/2, f_hat/1
  Sum4/1 -> convert virtual input u_x to desired theta/1(u_x)  "u_x = u_x0 + kd_h*n_hat_xdot - f_hat_x"
  phi/1 -> convert virtual input u_x to desired theta/4(phi)
  m/1 -> convert virtual input u_x to desired theta/2(m)
  psi/1 -> convert virtual input u_x to desired theta/5(psi)
  x_g_d_ddot/1 -> Sum/1
  x_g/1 -> NE_x/1(x_sensor), UDE_x/2(x_sensor (output1)), Sum1/2
  v_xg/1 -> NE_x/2(x_dot_sensor), UDE_x/3(x_dot_sensor (output2)), Sum2/2
  convert virtual input u_x to desired theta/1(theta_d) -> +-pi/8/1, Scope6/1
  UDE_x/1(f_hat_x) -> Manual Switch3/2
  T/1 -> convert virtual input u_x to desired theta/3(T)
  +-pi/8/1 -> Scope7/1, theta_d/1
  Gain2/1 -> Sum3/2
  UDE_x classic/1(f_hat_x) -> Manual Switch3/1
  2/1 -> Manual Switch2/2
  Manual Switch3/1 -> Manual Switch2/1

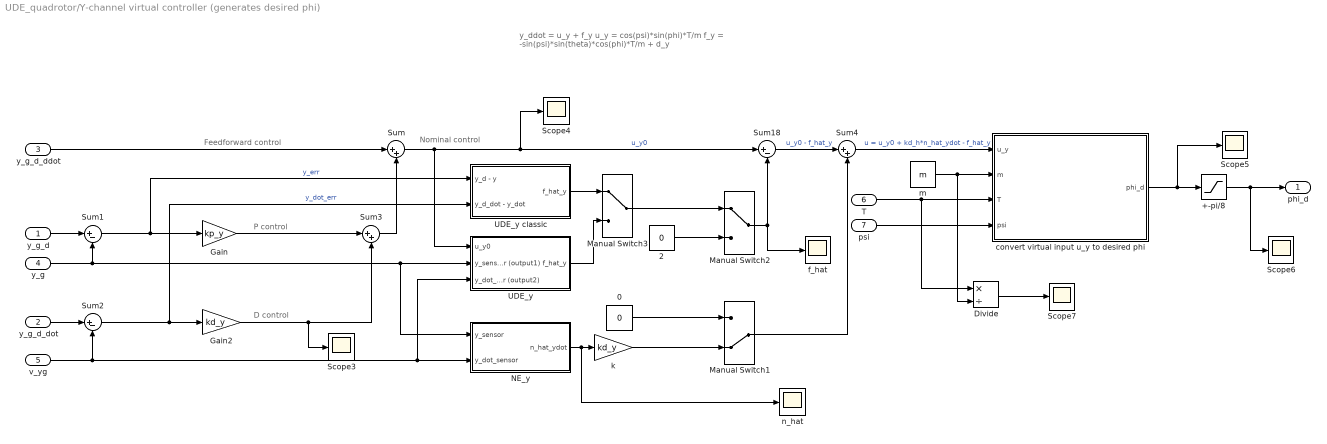
== system UDE_quadrotor/Y-channel virtual controller (generates desired phi) ==
  note: Nominal control
  note: Feedforward control
  note: D control
  note: y_ddot = u_y + f_y
      | u_y = cos(psi)*sin(phi)*T/m
      | f_y = -sin(psi)*sin(theta)*cos(phi)*T/m + d_y
  note: P control
  y_g_d : Inport
  y_g_d_dot : Inport  Port=2
  y_g_d_ddot : Inport  Port=3
  y_g : Inport  Port=4
  v_yg : Inport  Port=5
  T : Inport  Port=6
  psi : Inport  Port=7
  +-pi/8 : Saturate  UpperLimit=pi/8  LowerLimit=-pi/8
  0 : Constant  Value=0
  2 : Constant  Value=0
  Divide : Product  Inputs=*/
  Gain : Gain  Gain=kp_y
  Gain2 : Gain  Gain=kd_y
  Manual Switch1 : ManualSwitch  CurrentSetting=0
  Manual Switch2 : ManualSwitch
  Manual Switch3 : ManualSwitch
  NE_y : Subsystem
  Scope{3..7} (5 alike) : Scope
  Sum : Sum  Inputs=|++
  Sum1 : Sum  Inputs=|+-
  Sum18 : Sum  Inputs=|+-
  Sum2 : Sum  Inputs=|+-
  Sum3 : Sum  Inputs=|++
  Sum4 : Sum  Inputs=|++
  UDE_y : Subsystem
  UDE_y classic : Subsystem
  convert virtual input u_y to desired phi : MATLAB Function  TreatAsAtomicUnit=on
  f_hat : Scope
  k : Gain  Gain=kd_y
  m : Constant  Value=m
  n_hat : Scope
  phi_d : Outport
  wires:
  T/1 -> Divide/1, convert virtual input u_y to desired phi/3(T)
  UDE_y/1(f_hat_y) -> Manual Switch3/2
  convert virtual input u_y to desired phi/1(phi_d) -> Scope5/1, +-pi/8/1
  v_yg/1 -> Sum2/2, UDE_y/3(y_dot_sensor (output2)), NE_y/2(y_dot_sensor)
  y_g/1 -> Sum1/2, UDE_y/2(y_sensor (output1)), NE_y/1(y_sensor)
  y_g_d_ddot/1 -> Sum/1
  psi/1 -> convert virtual input u_y to desired phi/4(psi)
  m/1 -> Divide/2, convert virtual input u_y to desired phi/2(m)
  Sum4/1 -> convert virtual input u_y to desired phi/1(u_y)  "u = u_y0 + kd_h*n_hat_ydot - f_hat_y"
  Manual Switch2/1 -> Sum18/2, f_hat/1
  Manual Switch1/1 -> Sum4/2
  0/1 -> Manual Switch1/1
  NE_y/1(n_hat_ydot) -> k/1, n_hat/1
  k/1 -> Manual Switch1/2
  Sum18/1 -> Sum4/1  "u_y0 - f_hat_y"
  Gain2/1 -> Scope3/1, Sum3/2
  Sum2/1 -> UDE_y classic/2(y_d_dot - y_dot), Gain2/1  "y_dot_err"
  Sum1/1 -> UDE_y classic/1(y_d - y), Gain/1  "y_err"
  y_g_d/1 -> Sum1/1
  Sum/1 -> UDE_y/1(u_y0), Scope4/1, Sum18/1  "u_y0"
  Sum3/1 -> Sum/2
  y_g_d_dot/1 -> Sum2/1
  +-pi/8/1 -> Scope6/1, phi_d/1
  Gain/1 -> Sum3/1
  Divide/1 -> Scope7/1
  2/1 -> Manual Switch2/2
  UDE_y classic/1(f_hat_y) -> Manual Switch3/1
  Manual Switch3/1 -> Manual Switch2/1

== system UDE_quadrotor/Yaw (psi) controller ==
  note: setting psi_d_ddot to 0 means the nominal controller can not deliver asymptotic tracking of a time-varing psi angular rate reference
  note: psi_ddot = u_ psi + ftau_zb
      | u_ psi = psi _d_ddot + kp_ psi *( psi _d- psi ) + pd_ psi *( psi _d_dot - psi _dot) - ftau_zb_hat
      | ftau_zb_hat = - (1/T_psi) * [kd_ psi *( psi _d - psi ) + kp_ psi * integral( psi _d - psi ) + ( psi _d_dot - psi _dot)]
  psi_d : Inport
  psi_d_dot : Inport  Port=2
  psi_d_ddot : Inport  Port=3
  psi : Inport  Port=4
  psi_dot : Inport  Port=5
  Gain : Gain  Gain=kp_psi
  Gain4 : Gain  Gain=kd_psi
  Saturation : Saturate  UpperLimit=tau_z_max  LowerLimit=-tau_z_max
  Sum1 : Sum  Inputs=|+-
  Sum2 : Sum  Inputs=|+-
  Sum3 : Sum  Inputs=|++
  Sum4 : Sum  Inputs=|+-
  Sum5 : Sum  Inputs=++|
  UDE_psi : Subsystem
  tau_z_cmd : Outport
  wires:
  psi_d_dot/1 -> Sum2/1
  Gain4/1 -> Sum3/2
  Sum4/1 -> Saturation/1
  UDE_psi/1(ftau_yb_hat) -> Sum4/2
  psi/1 -> Sum1/2
  Sum5/1 -> Sum4/1  "u_psi_0"
  Gain/1 -> Sum3/1
  psi_dot/1 -> Sum2/2
  psi_d/1 -> Sum1/1
  Sum3/1 -> Sum5/2
  Sum1/1 -> UDE_psi/1(theta_d - theta), Gain/1
  Sum2/1 -> UDE_psi/2(theta_d_dot - theta_dot), Gain4/1
  psi_d_ddot/1 -> Sum5/1
  Saturation/1 -> tau_z_cmd/1

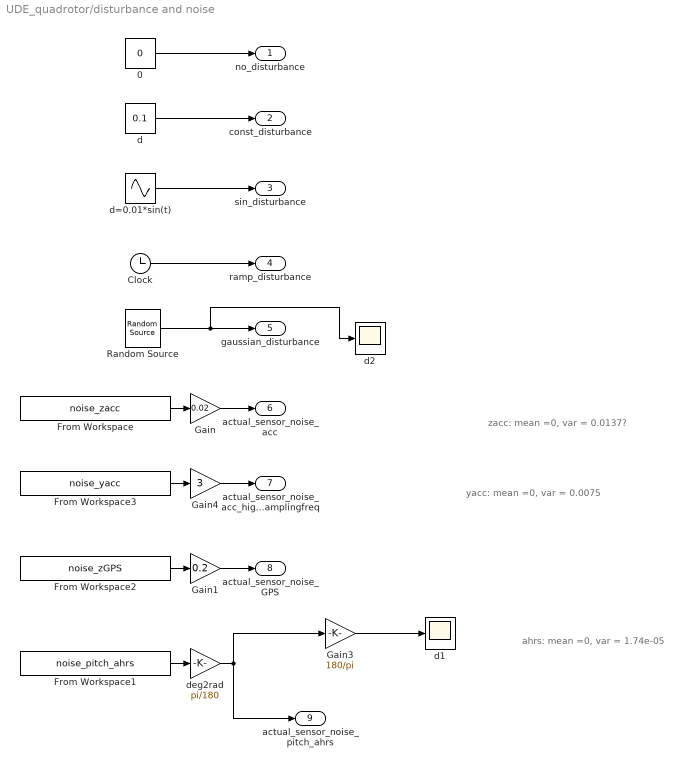
== system UDE_quadrotor/disturbance and noise ==
  note: ahrs: mean =0, var = 1.74e-05
  note: zacc: mean =0, var = 0.0137?
  note: yacc: mean =0, var = 0.0075
  0 : Constant  Value=0
  Clock : Clock
  From Workspace : FromWorkspace  VariableName=noise_zacc  OutputAfterFinalValue=Setting to zero
  From Workspace1 : FromWorkspace  VariableName=noise_pitch_ahrs  OutputAfterFinalValue=Setting to zero
  From Workspace2 : FromWorkspace  VariableName=noise_zGPS  OutputAfterFinalValue=Setting to zero
  From Workspace3 : FromWorkspace  VariableName=noise_yacc  OutputAfterFinalValue=Setting to zero
  Gain : Gain  Gain=0.02
  Gain1 : Gain  Gain=0.2
  Gain3 : Gain  Gain=180/pi
  Gain4 : Gain  Gain=3
  Random Source : dspsrcs4/Random Source  SrcType=Gaussian  NormMethod=Ziggurat  CltLength=12  MinVal=0  MaxVal=1  MeanVal=0  VarVal=0.02  RepMode=Repeatable  rawSeed=1  IsInherit=off  SampMode=Continuous  SampTime=1  SampFrame=1  DataType=Double  OutComplex=Real  OutputFrames=on
  d : Constant  Value=0.1
  d1 : Scope
  d2 : Scope
  d=0.01*sin(t) : Sin  Amplitude=0.01  SampleTime=0
  deg2rad : Gain  Gain=pi/180
  no_disturbance : Outport
  const_disturbance : Outport  Port=2
  sin_disturbance : Outport  Port=3
  ramp_disturbance : Outport  Port=4
  gaussian_disturbance : Outport  Port=5
  actual_sensor_noise_acc : Outport  Port=6
  actual_sensor_noise_acc_highsamplingfreq : Outport  Port=7
  actual_sensor_noise_GPS : Outport  Port=8
  actual_sensor_noise_pitch_ahrs : Outport  Port=9
  wires:
  d/1 -> const_disturbance/1
  d=0.01*sin(t)/1 -> sin_disturbance/1
  Clock/1 -> ramp_disturbance/1
  From Workspace/1 -> Gain/1
  Gain/1 -> actual_sensor_noise_acc/1
  Random Source/1 -> d2/1, gaussian_disturbance/1
  From Workspace2/1 -> Gain1/1
  Gain1/1 -> actual_sensor_noise_GPS/1
  0/1 -> no_disturbance/1
  From Workspace1/1 -> deg2rad/1
  From Workspace3/1 -> Gain4/1
  Gain4/1 -> actual_sensor_noise_acc_highsamplingfreq/1
  deg2rad/1 -> Gain3/1, actual_sensor_noise_pitch_ahrs/1
  Gain3/1 -> d1/1

== system UDE_quadrotor/Height controller/NE_h ==
  h_sensor : Inport
  h_dot_sensor : Inport  Port=2
  Constant : Constant  Value=0
  Sum : Sum  Inputs=|++
  Sum2 : Sum  Inputs=|+-
  TF1 : TransferFcn  Denominator=[Tn_h 1]
  TF2 : TransferFcn  Numerator=[1 0]  Denominator=[Tn_h 1]
  TF3 : TransferFcn  Numerator=[1 0]  Denominator=[Tn_h 1]
  h_sensor(0) : Integrator  InitialConditionSource=external
  n_hat_hdot : Outport
  wires:
  h_sensor/1 -> TF2/1, h_sensor(0)/2
  Sum2/1 -> n_hat_hdot/1
  TF2/1 -> Sum2/2
  TF1/1 -> Sum/1
  Constant/1 -> h_sensor(0)/1
  h_sensor(0)/1 -> TF3/1
  h_dot_sensor/1 -> TF1/1
  Sum/1 -> Sum2/1
  TF3/1 -> Sum/2  "y1(0)/s  *  s/(Tn*s+1) = y1(0)/(Tn*s+1)"

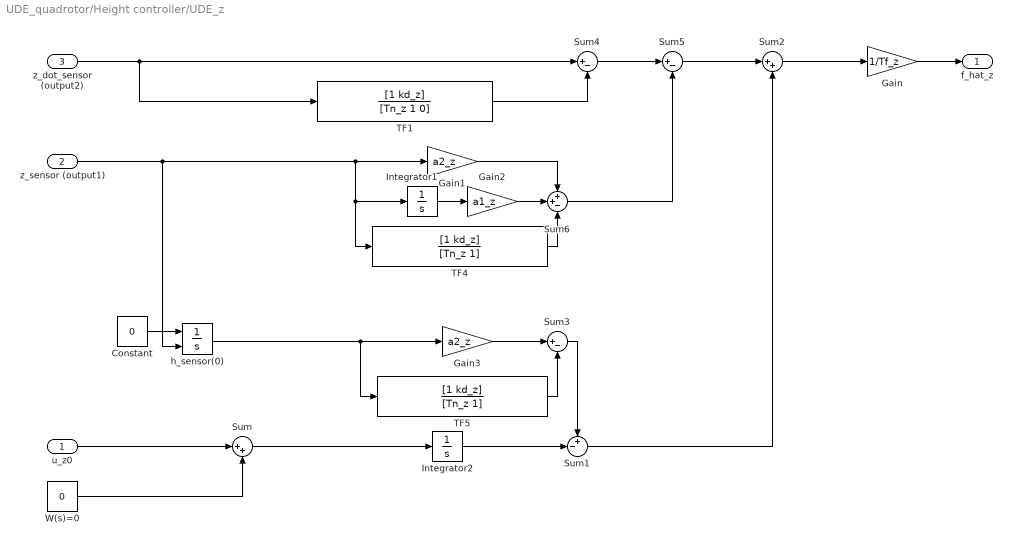
== system UDE_quadrotor/Height controller/UDE_z ==
  u_z0 : Inport
  z_sensor (output1) : Inport  Port=2
  z_dot_sensor (output2) : Inport  Port=3
  Constant : Constant  Value=0
  Gain : Gain  Gain=1/Tf_z
  Gain1 : Gain  Gain=a2_z
  Gain2 : Gain  Gain=a1_z
  Gain3 : Gain  Gain=a2_z
  Integrator1 : Integrator
  Integrator2 : Integrator
  Sum : Sum  Inputs=|++
  Sum1 : Sum  Inputs=+-|
  Sum2 : Sum  Inputs=|++
  Sum3 : Sum  Inputs=|+-
  Sum4 : Sum  Inputs=|+-
  Sum5 : Sum  Inputs=|+-
  Sum6 : Sum  Inputs=++-
  TF1 : TransferFcn  Numerator=[1 kd_z]  Denominator=[Tn_z 1 0]
  TF4 : TransferFcn  Numerator=[1 kd_z]  Denominator=[Tn_z 1]
  TF5 : TransferFcn  Numerator=[1 kd_z]  Denominator=[Tn_z 1]
  W(s)=0 : Constant  Value=0
  h_sensor(0) : Integrator  InitialConditionSource=external
  f_hat_z : Outport
  wires:
  Sum/1 -> Integrator2/1
  u_z0/1 -> Sum/1
  Gain/1 -> f_hat_z/1
  h_sensor(0)/1 -> TF5/1, Gain3/1
  Constant/1 -> h_sensor(0)/1
  z_sensor (output1)/1 -> Gain1/1, TF4/1, Integrator1/1, h_sensor(0)/2
  z_dot_sensor (output2)/1 -> Sum4/1, TF1/1
  W(s)=0/1 -> Sum/2
  Sum2/1 -> Gain/1
  TF1/1 -> Sum4/2
  Sum4/1 -> Sum5/1
  Gain1/1 -> Sum6/1
  Integrator1/1 -> Gain2/1
  Gain2/1 -> Sum6/2
  Sum6/1 -> Sum5/2
  TF4/1 -> Sum6/3
  Sum5/1 -> Sum2/1
  Sum1/1 -> Sum2/2
  Gain3/1 -> Sum3/1
  TF5/1 -> Sum3/2
  Sum3/1 -> Sum1/1
  Integrator2/1 -> Sum1/2

== system UDE_quadrotor/Height controller/UDE_z classic ==
  z_d - z : Inport
  z_d_dot - z_dot : Inport  Port=2
  Gain1 : Gain  Gain=kd_z
  Gain2 : Gain  Gain=-1/T_z
  Gain3 : Gain  Gain=kp_z
  Integrator : Integrator
  Sum6 : Sum  Inputs=+++
  f_hat_z : Outport
  wires:
  z_d - z/1 -> Integrator/1, Gain1/1
  Integrator/1 -> Gain3/1
  Gain1/1 -> Sum6/1
  Sum6/1 -> Gain2/1
  Gain3/1 -> Sum6/2
  Gain2/1 -> f_hat_z/1
  z_d_dot - z_dot/1 -> Sum6/3

== system UDE_quadrotor/Motors & Propellers/Force ==
  Rotor_speed : Inport
  Gain : Gain  OutDataTypeStr=Inherit: Same as input
  Multiply : Product  OutDataTypeStr=Inherit: Same as first input
  Square : Math  Operator=square  OutDataTypeStr=double  SaturateOnIntegerOverflow=on
  Sum of Elements : Sum  Inputs=+  OutDataTypeStr=Inherit: Same as first input
  cT : Constant  Value=hT
  force_B_N : Outport
  wires:
  Multiply/1 -> Sum of Elements/1
  Square/1 -> Multiply/1
  cT/1 -> Multiply/2
  Rotor_speed/1 -> Square/1
  Gain/1 -> force_B_N/1
  Sum of Elements/1 -> Gain/1

== system UDE_quadrotor/Motors & Propellers/Gyroscopic_Torque ==
  Rotor_speed : Inport
  p : Inport  Port=2
  q : Inport  Port=3
  Add : Sum  Inputs=--++
  Constant : Constant  Value=0
  Demux : Demux
  Gain : Gain  Gain=-Ir
  Gain1 : Gain  Gain=Ir
  Multiply1 : Product
  Multiply2 : Product
  Mux : Mux  Inputs=3
  gyroscopic_torque : Outport
  wires:
  Add/1 -> Multiply2/1, Multiply1/1
  Demux/1 -> Add/1
  Multiply1/1 -> Gain/1
  Rotor_speed/1 -> Demux/1
  Demux/3 -> Add/3
  Demux/2 -> Add/2
  Demux/4 -> Add/4
  Multiply2/1 -> Gain1/1
  Gain1/1 -> Mux/2
  Mux/1 -> gyroscopic_torque/1
  Constant/1 -> Mux/3
  Gain/1 -> Mux/1
  p/1 -> Multiply2/2
  q/1 -> Multiply1/2

== system UDE_quadrotor/Motors & Propellers/Rotor_Generated_Torque ==
  Rotor_speed : Inport
  Multiply1 : Product  Multiplication=Matrix(*)
  Square1 : Math  Operator=square  SaturateOnIntegerOverflow=on
  X_Frame : Constant  Value=[-LT*hT,LT*hT,LT*hT,-LT*hT;LT*hT,-LT*hT,LT*hT,-LT*hT;hM,hM,-hM,-hM]  OutDataTypeStr=double
  Torque : Outport
  wires:
  Square1/1 -> Multiply1/2
  Multiply1/1 -> Torque/1
  X_Frame/1 -> Multiply1/1
  Rotor_speed/1 -> Square1/1

== system UDE_quadrotor/Pitch (theta) controller/UDE_theta ==
  note: ftau_yb_hat = - (1/T_theta) * [kd_theta*(theta_d - theta) + kp_theta * integral(theta_d - theta) + (theta_d_dot - theta_dot)]
  theta_d - theta : Inport
  theta_d_dot - theta_dot : Inport  Port=2
  Gain1 : Gain  Gain=kd_theta
  Gain2 : Gain  Gain=-1/T_theta
  Gain3 : Gain  Gain=kp_theta
  Integrator : Integrator
  Sum6 : Sum  Inputs=+++
  ftau_yb_hat : Outport
  wires:
  theta_d_dot - theta_dot/1 -> Sum6/3
  theta_d - theta/1 -> Integrator/1, Gain1/1
  Integrator/1 -> Gain3/1
  Gain1/1 -> Sum6/1
  Sum6/1 -> Gain2/1
  Gain3/1 -> Sum6/2
  Gain2/1 -> ftau_yb_hat/1

== system UDE_quadrotor/Pitch (theta) controller/UDE_theta type1 (no velocity used) ==
  note: ftau_yb_hat = [s*theta(s) - theta (0)]/(T_ theta 1*s + T_ theta 2) - kp_ theta *[ theta _d(s) - theta (s)]/(T_ theta 1*s^2 + T_ theta 2*s) - kd_ theta *[ theta _d(s) - theta (s)]/[(T_ theta 1*s + T_ theta 2)*(T*s + 1)]
  theta_d - theta : Inport
  theta : Inport  Port=2
  Constant : Constant  Value=0
  Gain : Gain  Gain=kp_theta
  Gain4 : Gain  Gain=kd_theta
  Integrator : Integrator  InitialConditionSource=external
  Sum1 : Sum  Inputs=|+-
  Sum2 : Sum  Inputs=|+-
  Sum3 : Sum  Inputs=|+-
  Transfer Fcn : TransferFcn  Numerator=[1 0]  Denominator=[T_theta1 T_theta2]
  Transfer Fcn1 : TransferFcn  Numerator=[1 0]  Denominator=[T_theta1 T_theta2]
  Transfer Fcn2 : TransferFcn  Denominator=[T_theta1 T_theta2 0]
  Transfer Fcn3 : TransferFcn  Denominator=[T_theta1 T_theta2]
  Transfer Fcn4 : TransferFcn  Denominator=[T_passive 1]
  ftau_yb_hat : Outport
  wires:
  theta/1 -> Integrator/2, Transfer Fcn/1
  Constant/1 -> Integrator/1
  Integrator/1 -> Transfer Fcn1/1  "theta(0)"
  Transfer Fcn/1 -> Sum1/1
  Transfer Fcn1/1 -> Sum1/2
  Sum1/1 -> Sum2/1
  Transfer Fcn2/1 -> Gain/1
  theta_d - theta/1 -> Transfer Fcn3/1, Transfer Fcn2/1
  Sum2/1 -> Sum3/1
  Gain/1 -> Sum2/2
  Transfer Fcn3/1 -> Transfer Fcn4/1
  Transfer Fcn4/1 -> Gain4/1
  Gain4/1 -> Sum3/2
  Sum3/1 -> ftau_yb_hat/1

== system UDE_quadrotor/Pitch (theta) controller/UDE_theta type2 (no desired velocity used) ==
  note: ftau_yb_hat = 1/T_theta*[theta_dot(s) - theta_dot(0)/s - kp_theta*(theta_d(s)-theta(s))/s - kd_theta*(theta_d(s)-theta(s))/(T_passive+1)]
  theta_d - theta : Inport
  theta_dot : Inport  Port=2
  Constant : Constant  Value=0
  Gain : Gain  Gain=kp_theta
  Gain2 : Gain  Gain=1/T_theta3
  Gain4 : Gain  Gain=kd_theta
  Integrator : Integrator  InitialConditionSource=external
  Integrator1 : Integrator
  Sum1 : Sum  Inputs=|+-
  Sum2 : Sum  Inputs=|+-
  Sum3 : Sum  Inputs=|+-
  Transfer Fcn4 : TransferFcn  Denominator=[T_passive 1]
  ftau_yb_hat : Outport
  wires:
  Constant/1 -> Integrator/1
  Integrator/1 -> Sum1/2  "theta_dot(0)"
  theta_dot/1 -> Sum1/1, Integrator/2
  Sum1/1 -> Sum2/1
  Integrator1/1 -> Gain/1
  Sum2/1 -> Sum3/1
  Gain/1 -> Sum2/2
  theta_d - theta/1 -> Transfer Fcn4/1, Integrator1/1
  Transfer Fcn4/1 -> Gain4/1
  Gain4/1 -> Sum3/2
  Sum3/1 -> Gain2/1
  Gain2/1 -> ftau_yb_hat/1

== system UDE_quadrotor/Roll (phi) controller/UDE_phi ==
  note: ftau_xb_hat = - (1/T_phi) * [kd_phi*(phi_d - phi) + kp_phi * integral(phi_d - phi) + (phi_d_dot - phi_dot)]
  phi_d - phi : Inport
  phi_d_dot - phi_dot : Inport  Port=2
  Gain1 : Gain  Gain=kd_phi
  Gain2 : Gain  Gain=-1/T_phi
  Gain3 : Gain  Gain=kp_phi
  Integrator : Integrator
  Sum6 : Sum  Inputs=+++
  ftau_xb_hat : Outport
  wires:
  phi_d - phi/1 -> Integrator/1, Gain1/1
  Integrator/1 -> Gain3/1
  Gain1/1 -> Sum6/1
  Sum6/1 -> Gain2/1
  Gain3/1 -> Sum6/2
  Gain2/1 -> ftau_xb_hat/1
  phi_d_dot - phi_dot/1 -> Sum6/3

== system UDE_quadrotor/Roll (phi) controller/UDE_phi type1 (no velocity used) ==
  note: ftau_xb_hat = [s*phi(s) - phi(0)]/(T_phi1*s + T_phi2) - kp_phi*[phi_d(s) - phi(s)]/(T_phi1*s^2 + T_phi2*s) - kd_phi*[phi_d(s) - phi(s)]/[(T_phi1*s + T_phi2)*(T*s + 1)]
  phi_d - phi : Inport
  phi : Inport  Port=2
  Constant : Constant  Value=0
  Gain : Gain  Gain=kp_phi
  Gain4 : Gain  Gain=kd_phi
  Integrator : Integrator  InitialConditionSource=external
  Sum1 : Sum  Inputs=|+-
  Sum2 : Sum  Inputs=|+-
  Sum3 : Sum  Inputs=|+-
  Transfer Fcn : TransferFcn  Numerator=[1 0]  Denominator=[T_phi1 T_phi2]
  Transfer Fcn1 : TransferFcn  Numerator=[1 0]  Denominator=[T_phi1 T_phi2]
  Transfer Fcn2 : TransferFcn  Denominator=[T_phi1 T_phi2 0]
  Transfer Fcn3 : TransferFcn  Denominator=[T_phi1 T_phi2]
  Transfer Fcn5 : TransferFcn  Denominator=[T_passive 1]
  ftau_xb_hat : Outport
  wires:
  phi/1 -> Integrator/2, Transfer Fcn/1
  Constant/1 -> Integrator/1
  Integrator/1 -> Transfer Fcn1/1  "phi(0)"
  Transfer Fcn/1 -> Sum1/1
  Transfer Fcn1/1 -> Sum1/2
  Sum1/1 -> Sum2/1
  Transfer Fcn2/1 -> Gain/1
  phi_d - phi/1 -> Transfer Fcn3/1, Transfer Fcn2/1
  Sum2/1 -> Sum3/1
  Gain/1 -> Sum2/2
  Transfer Fcn3/1 -> Transfer Fcn5/1
  Transfer Fcn5/1 -> Gain4/1
  Gain4/1 -> Sum3/2
  Sum3/1 -> ftau_xb_hat/1

== system UDE_quadrotor/Roll (phi) controller/UDE_phi type2 (no desired velocity used) ==
  note: ftau_xb_hat = 1/T_phi*[phi_dot(s) - phi_dot(0)/s - kp_phi*(phi_d(s)-phi(s))/s - kd_phi*(phi_d(s)-phi(s))/(T_passive+1)]
  phi_d - phi : Inport
  phi_dot : Inport  Port=2
  Constant : Constant  Value=0
  Gain : Gain  Gain=kp_phi
  Gain2 : Gain  Gain=1/T_phi3
  Gain4 : Gain  Gain=kd_phi
  Integrator : Integrator  InitialConditionSource=external
  Integrator1 : Integrator
  Sum1 : Sum  Inputs=|+-
  Sum2 : Sum  Inputs=|+-
  Sum3 : Sum  Inputs=|+-
  Transfer Fcn4 : TransferFcn  Denominator=[T_passive 1]
  ftau_xb_hat : Outport
  wires:
  Constant/1 -> Integrator/1
  Integrator/1 -> Sum1/2  "phi_dot(0)"
  phi_dot/1 -> Sum1/1, Integrator/2
  Sum1/1 -> Sum2/1
  Integrator1/1 -> Gain/1
  Sum2/1 -> Sum3/1
  Gain/1 -> Sum2/2
  phi_d - phi/1 -> Transfer Fcn4/1, Integrator1/1
  Transfer Fcn4/1 -> Gain4/1
  Gain4/1 -> Sum3/2
  Sum3/1 -> Gain2/1
  Gain2/1 -> ftau_xb_hat/1

== system UDE_quadrotor/X-channel virtual controller (generates desired theta)/NE_x ==
  x_sensor : Inport
  x_dot_sensor : Inport  Port=2
  Constant : Constant  Value=0
  Sum : Sum  Inputs=|++
  Sum2 : Sum  Inputs=|+-
  TF1 : TransferFcn  Denominator=[Tn_x 1]
  TF2 : TransferFcn  Numerator=[1 0]  Denominator=[Tn_x 1]
  TF3 : TransferFcn  Numerator=[1 0]  Denominator=[Tn_x 1]
  x_sensor(0) : Integrator  InitialConditionSource=external
  n_hat_xdot : Outport
  wires:
  x_sensor/1 -> TF2/1, x_sensor(0)/2
  Sum2/1 -> n_hat_xdot/1
  TF2/1 -> Sum2/2
  TF1/1 -> Sum/1
  Constant/1 -> x_sensor(0)/1
  x_sensor(0)/1 -> TF3/1
  x_dot_sensor/1 -> TF1/1
  Sum/1 -> Sum2/1
  TF3/1 -> Sum/2  "y1(0)/s  *  s/(Tn*s+1) = y1(0)/(Tn*s+1)"

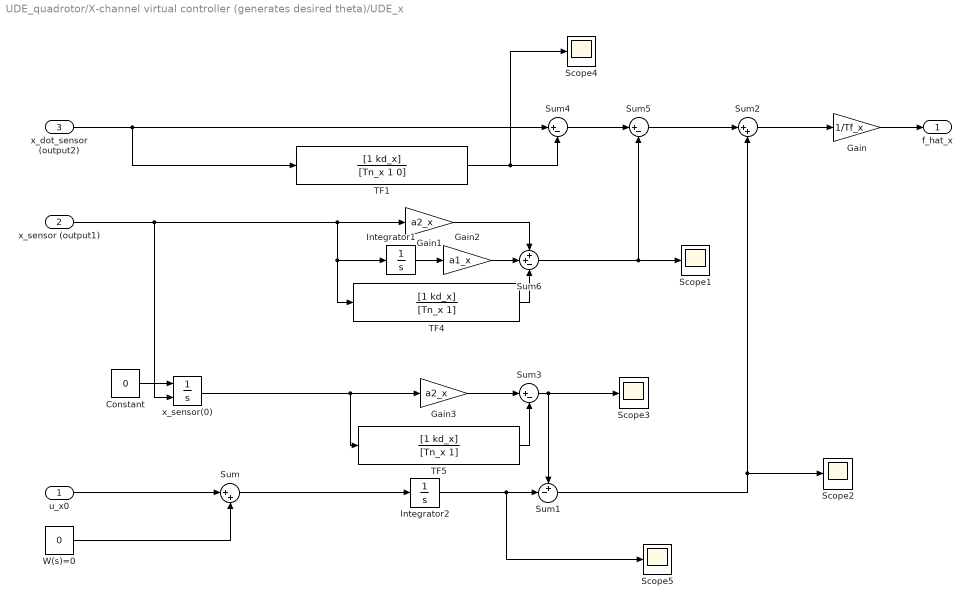
== system UDE_quadrotor/X-channel virtual controller (generates desired theta)/UDE_x ==
  u_x0 : Inport
  x_sensor (output1) : Inport  Port=2
  x_dot_sensor (output2) : Inport  Port=3
  Constant : Constant  Value=0
  Gain : Gain  Gain=1/Tf_x
  Gain1 : Gain  Gain=a2_x
  Gain2 : Gain  Gain=a1_x
  Gain3 : Gain  Gain=a2_x
  Integrator1 : Integrator
  Integrator2 : Integrator
  Scope{1..5} (5 alike) : Scope
  Sum : Sum  Inputs=|++
  Sum1 : Sum  Inputs=+-|
  Sum2 : Sum  Inputs=|++
  Sum3 : Sum  Inputs=|+-
  Sum4 : Sum  Inputs=|+-
  Sum5 : Sum  Inputs=|+-
  Sum6 : Sum  Inputs=++-
  TF1 : TransferFcn  Numerator=[1 kd_x]  Denominator=[Tn_x 1 0]
  TF4 : TransferFcn  Numerator=[1 kd_x]  Denominator=[Tn_x 1]
  TF5 : TransferFcn  Numerator=[1 kd_x]  Denominator=[Tn_x 1]
  W(s)=0 : Constant  Value=0
  x_sensor(0) : Integrator  InitialConditionSource=external
  f_hat_x : Outport
  wires:
  Sum/1 -> Integrator2/1
  u_x0/1 -> Sum/1
  Gain/1 -> f_hat_x/1
  x_sensor(0)/1 -> TF5/1, Gain3/1
  Constant/1 -> x_sensor(0)/1
  x_sensor (output1)/1 -> Gain1/1, TF4/1, Integrator1/1, x_sensor(0)/2
  x_dot_sensor (output2)/1 -> Sum4/1, TF1/1
  W(s)=0/1 -> Sum/2
  Sum2/1 -> Gain/1
  Sum4/1 -> Sum5/1
  Gain1/1 -> Sum6/1
  Integrator1/1 -> Gain2/1
  Gain2/1 -> Sum6/2
  Sum6/1 -> Scope1/1, Sum5/2
  TF4/1 -> Sum6/3
  Sum5/1 -> Sum2/1
  Sum1/1 -> Scope2/1, Sum2/2
  Gain3/1 -> Sum3/1
  TF5/1 -> Sum3/2
  Sum3/1 -> Scope3/1, Sum1/1
  Integrator2/1 -> Scope5/1, Sum1/2
  TF1/1 -> Scope4/1, Sum4/2

== system UDE_quadrotor/X-channel virtual controller (generates desired theta)/UDE_x classic ==
  x_d - x : Inport
  x_d_dot - x_dot : Inport  Port=2
  Gain1 : Gain  Gain=kd_x
  Gain2 : Gain  Gain=-1/T_x
  Gain3 : Gain  Gain=kp_x
  Integrator : Integrator
  Sum6 : Sum  Inputs=+++
  f_hat_x : Outport
  wires:
  x_d - x/1 -> Integrator/1, Gain1/1
  Integrator/1 -> Gain3/1
  Gain1/1 -> Sum6/1
  Sum6/1 -> Gain2/1
  Gain3/1 -> Sum6/2
  Gain2/1 -> f_hat_x/1
  x_d_dot - x_dot/1 -> Sum6/3

== system UDE_quadrotor/Y-channel virtual controller (generates desired phi)/NE_y ==
  y_sensor : Inport
  y_dot_sensor : Inport  Port=2
  Constant : Constant  Value=0
  Sum : Sum  Inputs=|++
  Sum2 : Sum  Inputs=|+-
  TF1 : TransferFcn  Denominator=[Tn_y 1]
  TF2 : TransferFcn  Numerator=[1 0]  Denominator=[Tn_y 1]
  TF3 : TransferFcn  Numerator=[1 0]  Denominator=[Tn_y 1]
  y_sensor(0) : Integrator  InitialConditionSource=external
  n_hat_ydot : Outport
  wires:
  TF3/1 -> Sum/2  "y1(0)/s  *  s/(Tn*s+1) = y1(0)/(Tn*s+1)"
  Sum/1 -> Sum2/1
  y_dot_sensor/1 -> TF1/1
  y_sensor(0)/1 -> TF3/1
  Constant/1 -> y_sensor(0)/1
  TF1/1 -> Sum/1
  TF2/1 -> Sum2/2
  Sum2/1 -> n_hat_ydot/1
  y_sensor/1 -> y_sensor(0)/2, TF2/1

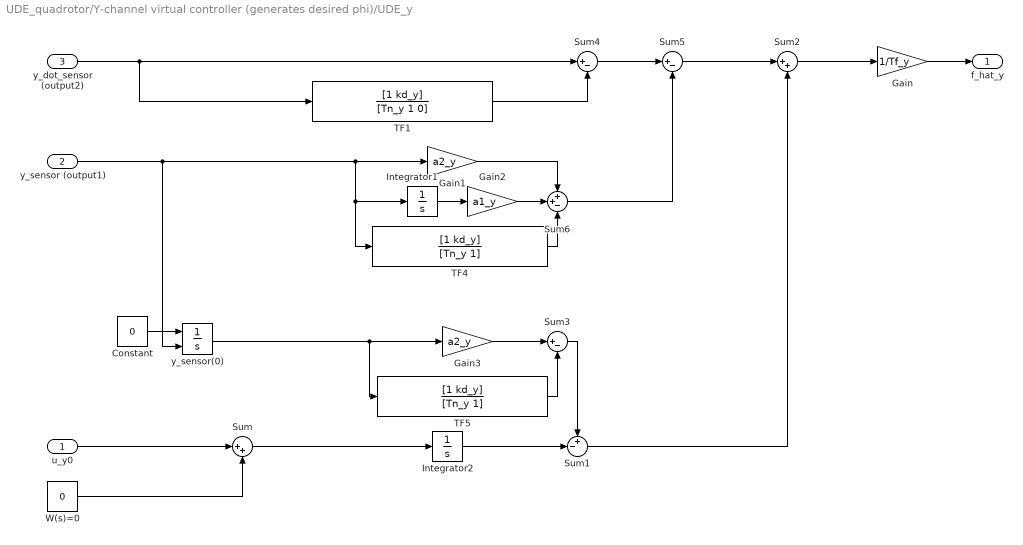
== system UDE_quadrotor/Y-channel virtual controller (generates desired phi)/UDE_y ==
  u_y0 : Inport
  y_sensor (output1) : Inport  Port=2
  y_dot_sensor (output2) : Inport  Port=3
  Constant : Constant  Value=0
  Gain : Gain  Gain=1/Tf_y
  Gain1 : Gain  Gain=a2_y
  Gain2 : Gain  Gain=a1_y
  Gain3 : Gain  Gain=a2_y
  Integrator1 : Integrator
  Integrator2 : Integrator
  Sum : Sum  Inputs=|++
  Sum1 : Sum  Inputs=+-|
  Sum2 : Sum  Inputs=|++
  Sum3 : Sum  Inputs=|+-
  Sum4 : Sum  Inputs=|+-
  Sum5 : Sum  Inputs=|+-
  Sum6 : Sum  Inputs=++-
  TF1 : TransferFcn  Numerator=[1 kd_y]  Denominator=[Tn_y 1 0]
  TF4 : TransferFcn  Numerator=[1 kd_y]  Denominator=[Tn_y 1]
  TF5 : TransferFcn  Numerator=[1 kd_y]  Denominator=[Tn_y 1]
  W(s)=0 : Constant  Value=0
  y_sensor(0) : Integrator  InitialConditionSource=external
  f_hat_y : Outport
  wires:
  Integrator2/1 -> Sum1/2
  Sum3/1 -> Sum1/1
  TF5/1 -> Sum3/2
  Gain3/1 -> Sum3/1
  Sum1/1 -> Sum2/2
  Sum5/1 -> Sum2/1
  TF4/1 -> Sum6/3
  Sum6/1 -> Sum5/2
  Gain2/1 -> Sum6/2
  Integrator1/1 -> Gain2/1
  Gain1/1 -> Sum6/1
  Sum4/1 -> Sum5/1
  TF1/1 -> Sum4/2
  Sum2/1 -> Gain/1
  W(s)=0/1 -> Sum/2
  y_dot_sensor (output2)/1 -> TF1/1, Sum4/1
  y_sensor (output1)/1 -> y_sensor(0)/2, Integrator1/1, TF4/1, Gain1/1
  Constant/1 -> y_sensor(0)/1
  y_sensor(0)/1 -> Gain3/1, TF5/1
  Gain/1 -> f_hat_y/1
  u_y0/1 -> Sum/1
  Sum/1 -> Integrator2/1
